simulink model "HW_sim_2"  (R2019b)
settings: Solver=VariableStepAuto  StartTime=0.0  StopTime=60  RelTol=1e-3
values from neighbouring files (symbols this model uses):
  d0 = 8    [HW1_main.m]
  Kd_err = 0.2    [HW1_main.m]
  Kv = 0.5    [HW1_main.m]
  Kv_r = 0.4    [HW1_main.m]
  th_tar = 1    [HW1_main.m]
  v_tar = 36    [HW1_main.m]
  vh0 = 28    [HW1_main.m]
  vl0 = 36    [HW1_main.m]
  xh0 = 0    [HW1_main.m]
  xl0 = 50    [HW1_main.m]
undefined symbols (not defined in the file or in its folder): sigbuilder_block
libraries: cstblocks x2
settings Model: Creator=user  LastModifiedBy=user

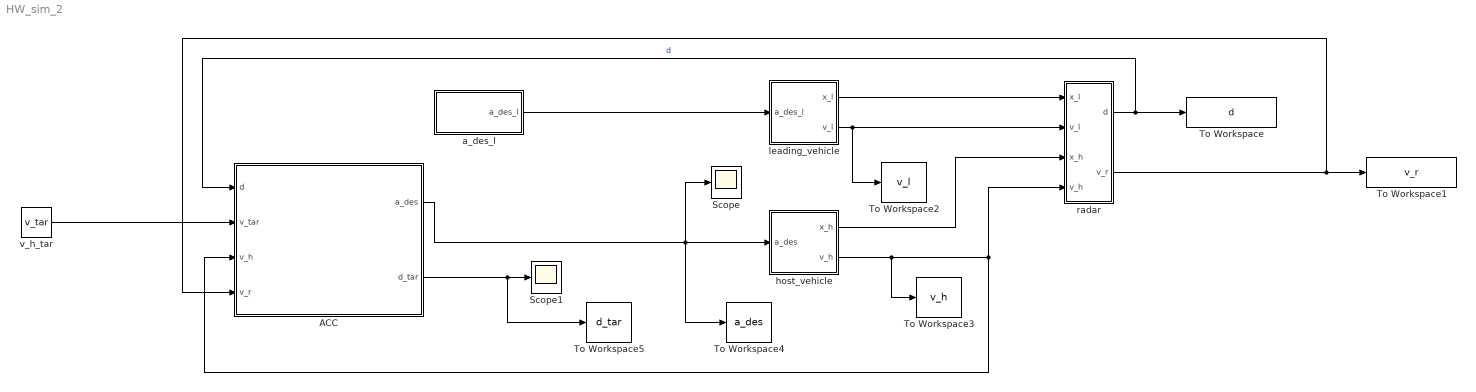
== system HW_sim_2 ==
  ACC : Subsystem
  Scope : Scope
  Scope1 : Scope
  To Workspace : ToWorkspace  VariableName=d  SaveFormat=Timeseries  SampleTime=-1
  To Workspace1 : ToWorkspace  VariableName=v_r  SaveFormat=Timeseries  SampleTime=-1
  To Workspace2 : ToWorkspace  VariableName=v_l  SaveFormat=Timeseries  SampleTime=-1
  To Workspace3 : ToWorkspace  VariableName=v_h  SaveFormat=Timeseries  SampleTime=-1
  To Workspace4 : ToWorkspace  VariableName=a_des  SaveFormat=Timeseries  SampleTime=-1
  To Workspace5 : ToWorkspace  VariableName=d_tar  SaveFormat=Timeseries  SampleTime=-1
  a_des_l : Subsystem  Tag=STV Subsys  LoadFcn=sigbuilder_block('load');  StartFcn=sigbuilder_block('start');  StopFcn=sigbuilder_block('stop');  ClipboardFcn=sigbuilder_block('clipboard');  mask(Sigbuilder block){tuvar=[0:10]}
      mask help: Simulink:masks:SigbuilderBlock_MD
      mask init:
      | if ~strcmp(get_param(bdroot(gcbh),'SimulationStatus'),'stopped') tuvar = sigbuilder_block('maskInit'); end
      settings: CopyFcn=sigbuilder_block('copy');  DeleteFcn=sigbuilder_block('delete');  ModelCloseFcn=sigbuilder_block('modelClose');  PreSaveFcn=sigbuilder_block('preSave');  PauseFcn=sigbuilder_block('pause');  ContinueFcn=sigbuilder_block('continue');  NameChangeFcn=sigbuilder_block('namechange');  OpenFcn=sigbuilder_block('open',[150 70 550.5 362.5 ]);  CloseFcn=sigbuilder_block('close');
      mask Display: plot(0, 0, 100, 100,[2, 2, 32, 32, 2], [68, 8, 8, 68, 68],[32, 2], [38, 38], [32, 19, 2],[53, 60, 44], [32, 17, 17, 2],[16, 16, 31, 31]);txt = getActiveGroup(gcbh);text(2, 100, txt,'verticalAlignment', 'top');
  host_vehicle : Subsystem
  leading_vehicle : Subsystem
  radar : Subsystem
  v_h_tar : Constant  Value=v_tar
  wires:
  leading_vehicle/1(x_l) -> radar/1(x_l)
  leading_vehicle/2(v_l) -> To Workspace2/1, radar/2(v_l)
  host_vehicle/1(x_h) -> radar/3(x_h)
  host_vehicle/2(v_h) -> To Workspace3/1, ACC/3(v_h), radar/4(v_h)
  ACC/1(a_des) -> host_vehicle/1(a_des), To Workspace4/1, Scope/1
  radar/2(v_r) -> ACC/4(v_r), To Workspace1/1
  radar/1(d) -> ACC/1(d), To Workspace/1  "d"
  v_h_tar/1 -> ACC/2(v_tar)
  a_des_l/1(a_des_l) -> leading_vehicle/1(a_des_l)
  ACC/2(d_tar) -> To Workspace5/1, Scope1/1

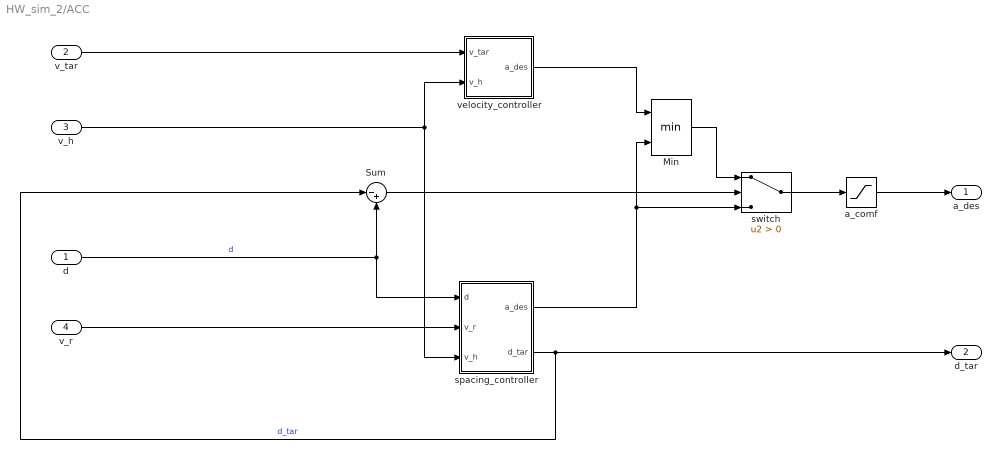
== system HW_sim_2/ACC ==
  d : Inport
  v_tar : Inport  Port=2
  v_h : Inport  Port=3
  v_r : Inport  Port=4
  Min : MinMax  Inputs=2
  Sum : Sum  Inputs=|-+
  a_comf : Saturate  UpperLimit=5  LowerLimit=-3
  spacing_controller : Subsystem
  switch : Switch  Criteria=u2 > Threshold
  velocity_controller : Subsystem
  a_des : Outport
  d_tar : Outport  Port=2
  wires:
  switch/1 -> a_comf/1
  spacing_controller/1(a_des) -> Min/2, switch/3
  Sum/1 -> switch/2
  d/1 -> Sum/2, spacing_controller/1(d)  "d"
  spacing_controller/2(d_tar) -> Sum/1, d_tar/1  "d_tar"
  v_r/1 -> spacing_controller/2(v_r)
  v_tar/1 -> velocity_controller/1(v_tar)
  v_h/1 -> spacing_controller/3(v_h), velocity_controller/2(v_h)
  a_comf/1 -> a_des/1
  Min/1 -> switch/1
  velocity_controller/1(a_des) -> Min/1

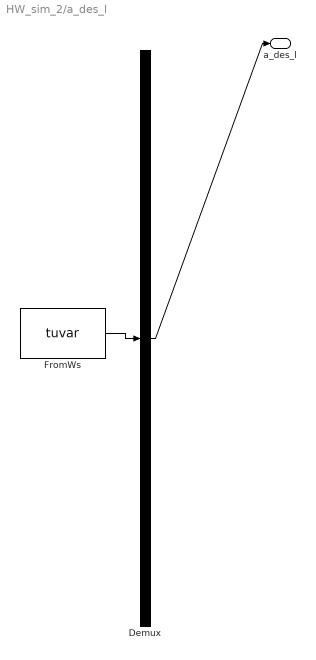
== system HW_sim_2/a_des_l ==
  Demux : Demux  Tag=STV Demux  Outputs=1
  FromWs : FromWorkspace  Tag=STV FromWs  VariableName=tuvar  SampleTime=0
      SigBuilderData=|
      | common.afterFinalStr = 'Extrapolate'
      | common.sampleTime = 0
      | dataSet.timeRange = [0 60]
      | dataSet.name = 'Group 1'
      | sbobj.Groups.Name = 'Group 1'
      | sbobj.Groups.Signals.Name = 'a_des_l'
      | sbobj.Groups.Signals.XData = [0 10 10.5 13.5 14 40 40.5 43.5 44 60]
      | sbobj.Groups.Signals.YData = [0 0 -2 -2 0 0 2 2 0 0]
      | sbobj.Groups.TimeRange = [0 60]
  a_des_l : Outport  Tag=STV Outport
  wires:
  FromWs/1 -> Demux/1
  Demux/1 -> a_des_l/1

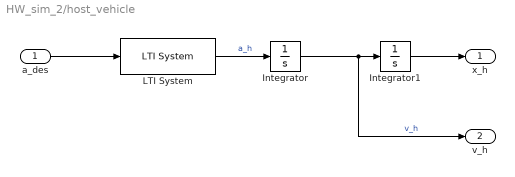
== system HW_sim_2/host_vehicle ==
  a_des : Inport
  Integrator : Integrator  InitialCondition=vh0
  Integrator1 : Integrator  InitialCondition=xh0
  LTI System : cstblocks/LTI System  sys=Gah  IC=[]
  x_h : Outport
  v_h : Outport  Port=2
  wires:
  LTI System/1 -> Integrator/1  "a_h"
  Integrator/1 -> v_h/1, Integrator1/1  "v_h"
  a_des/1 -> LTI System/1
  Integrator1/1 -> x_h/1

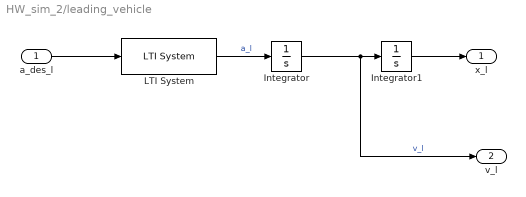
== system HW_sim_2/leading_vehicle ==
  a_des_l : Inport
  Integrator : Integrator  InitialCondition=vl0
  Integrator1 : Integrator  InitialCondition=xl0
  LTI System : cstblocks/LTI System  sys=Gah  IC=[]
  x_l : Outport
  v_l : Outport  Port=2
  wires:
  LTI System/1 -> Integrator/1  "a_l"
  Integrator/1 -> v_l/1, Integrator1/1  "v_l"
  a_des_l/1 -> LTI System/1
  Integrator1/1 -> x_l/1

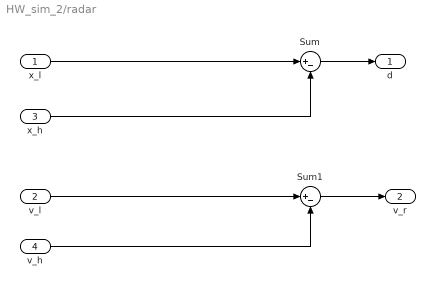
== system HW_sim_2/radar ==
  x_l : Inport
  v_l : Inport  Port=2
  x_h : Inport  Port=3
  v_h : Inport  Port=4
  Sum : Sum  Inputs=|+-
  Sum1 : Sum  Inputs=|+-
  d : Outport
  v_r : Outport  Port=2
  wires:
  x_l/1 -> Sum/1
  x_h/1 -> Sum/2
  v_l/1 -> Sum1/1
  Sum/1 -> d/1
  Sum1/1 -> v_r/1
  v_h/1 -> Sum1/2

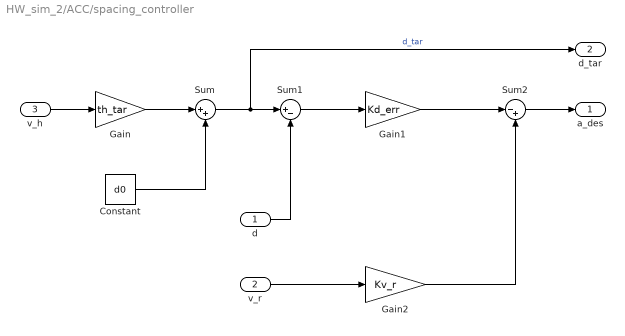
== system HW_sim_2/ACC/spacing_controller ==
  d : Inport
  v_r : Inport  Port=2
  v_h : Inport  Port=3
  Constant : Constant  Value=d0
  Gain : Gain  Gain=th_tar
  Gain1 : Gain  Gain=Kd_err
  Gain2 : Gain  Gain=Kv_r
  Sum : Sum  Inputs=|++
  Sum1 : Sum  Inputs=|+-
  Sum2 : Sum  Inputs=|-+
  a_des : Outport
  d_tar : Outport  Port=2
  wires:
  Gain/1 -> Sum/1
  v_r/1 -> Gain2/1
  Gain1/1 -> Sum2/1
  Sum/1 -> d_tar/1, Sum1/1  "d_tar"
  d/1 -> Sum1/2
  Constant/1 -> Sum/2
  v_h/1 -> Gain/1
  Sum2/1 -> a_des/1
  Gain2/1 -> Sum2/2
  Sum1/1 -> Gain1/1

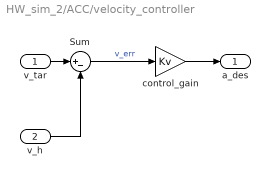
== system HW_sim_2/ACC/velocity_controller ==
  v_tar : Inport
  v_h : Inport  Port=2
  Sum : Sum  Inputs=|+-
  control_gain : Gain  Gain=Kv
  a_des : Outport
  wires:
  Sum/1 -> control_gain/1  "v_err"
  control_gain/1 -> a_des/1
  v_h/1 -> Sum/2
  v_tar/1 -> Sum/1
